simulink model "LC_core_control"  (R2023b)
settings: configuration reference "slow_tsk_conf" (kept outside this file)
settings Model: DataDictionary=fmuGenerationDictionay.sldd  Creator=Veimar  LastModifiedBy=Veimar
settings ConfigSetRef: SourceName=slow_tsk_conf

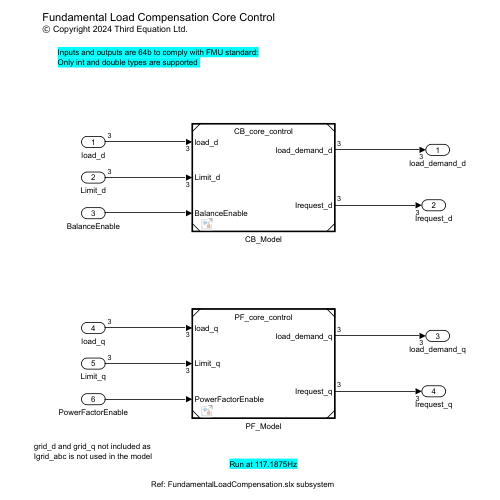
[thumbnail: Simulink's stored preview of the top-level diagram]
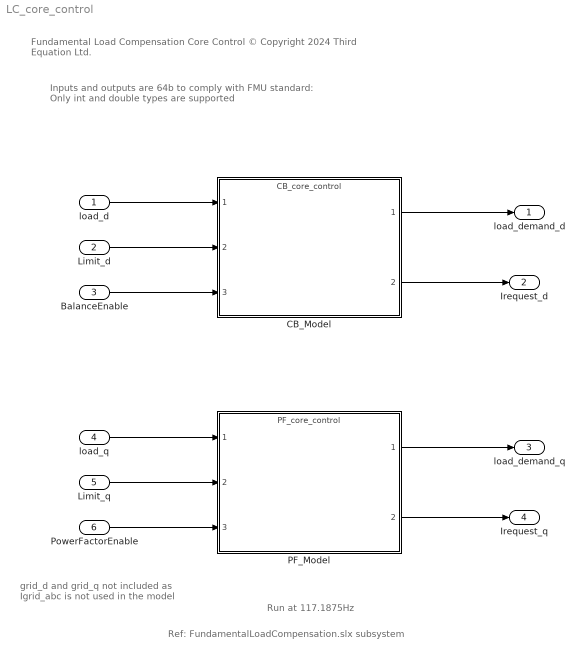
== system LC_core_control ==
  note: Fundamental Load Compensation Core Control
      | © Copyright 2024 Third Equation Ltd.
  note: Inputs and outputs are 64b to comply with FMU standard:
      | Only int and double types are supported
  note: Run at 117.1875Hz
  note: Ref: FundamentalLoadCompensation.slx subsystem
  note: grid_d and grid_q not included as
      | Igrid_abc is not used in the model
  load_d : Inport  OutDataTypeStr=single
  Limit_d : Inport  Port=2  OutDataTypeStr=single
  BalanceEnable : Inport  Port=3  OutDataTypeStr=boolean
  load_q : Inport  Port=4  OutDataTypeStr=single
  Limit_q : Inport  Port=5  OutDataTypeStr=single
  PowerFactorEnable : Inport  Port=6  OutDataTypeStr=boolean
  CB_Model : ModelReference  ModelNameDialog=CB_core_control.slx  SimulationMode=Normal  ModelReferenceVersion=1.44
  PF_Model : ModelReference  ModelNameDialog=PF_core_control.slx  SimulationMode=Normal  ModelReferenceVersion=1.43
  load_demand_d : Outport  OutDataTypeStr=single
  Irequest_d : Outport  Port=2  OutDataTypeStr=single
  load_demand_q : Outport  Port=3  OutDataTypeStr=single
  Irequest_q : Outport  Port=4  OutDataTypeStr=single
  wires:
  load_d/1 -> CB_Model/1
  Limit_d/1 -> CB_Model/2
  BalanceEnable/1 -> CB_Model/3
  CB_Model/1 -> load_demand_d/1
  CB_Model/2 -> Irequest_d/1
  PF_Model/2 -> Irequest_q/1
  PF_Model/1 -> load_demand_q/1
  Limit_q/1 -> PF_Model/2
  load_q/1 -> PF_Model/1
  PowerFactorEnable/1 -> PF_Model/3
